simulink model "verify_Valve_Thermostatic_mdl"  (R2016b)
settings: Solver=ode45  StartTime=0.0  StopTime=100  MaxStep=1  RelTol=1e-3  EnableMultiTasking=on
libraries: carnot x2, simulink x1
settings Model: Creator=drhf  LastModifiedBy=drhf
settings DataIOCC: SaveFormat=Array  SignalLoggingSaveFormat=ModelDataLogs
settings OptimizationCC: ExpressionDepthLimit=2147483647  LifeSpan=inf
settings DebuggingCC: UnderspecifiedInitializationDetection=Classic  MergeDetectMultiDrivingBlocksExec=none  SolverPrmCheckMsg=warning  FcnCallInpInsideContextMsg=warning  StateNameClashWarn=warning  SFUnexpectedBacktrackingDiag=warning  SFNoUnconditionalDefaultTransitionDiag=warning  SFExecutionAtInitializationDiag=none
settings HardwareCC: ProdBitPerPointer=32  ProdBitPerSizeT=32  ProdBitPerPtrDiffT=32  ProdLargestAtomicFloat=None  ProdIntDivRoundTo=Undefined  ProdEndianess=Unspecified  ProdWordSize=32  ProdHWDeviceType=32-bit Generic
settings ModelReferenceCC: PropagateSignalLabelsOutOfModel=off
settings GRTTargetCC: TargetLangStandard=C89/C90 (ANSI)  GeneratePreprocessorConditionals=Disable all  CombineOutputUpdateFcns=off  GRTInterface=on
settings ConfigComp: CovMetricSettings=dw  CovHtmlReporting=on  CovSaveCumulativeToWorkspaceVar=on  CovSaveSingleToWorkspaceVar=on  CovExternalEMLEnable=off

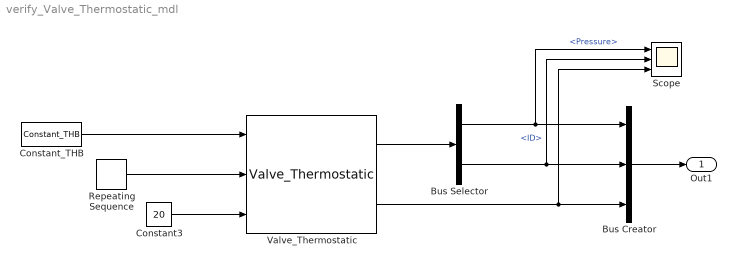
== system verify_Valve_Thermostatic_mdl ==
  Bus Creator : BusCreator  Inputs=3
  Bus Selector : BusSelector  OutputSignals=Pressure,ID
  Constant3 : Constant  Value=20
  Constant_THB : carnot/Source/Simple/Constant_THB  t=40  mdot=0.5  p=3e5  mID=Pressure Drop from Massflow  fluid=Water  mix=0  mix2=0  mix3=0  dia=0.02  hgt=0
  Repeating Sequence : simulink/Sources/Repeating Sequence  rep_seq_t=[0 50 100]  rep_seq_y=[15 25 15]
  Scope : Scope  NumInputPorts=3
  Valve_Thermostatic : carnot/Hydraulics/Valve_Thermostatic  p=4  op=0.5  bl=0.2  ts=1  dt_V=1  ART=linear  kvs=2  psi_0=0.04
  Out1 : Outport  SampleTime=5
  wires:
  Bus Creator/1 -> Out1/1
  Bus Selector/1 -> Bus Creator/1, Scope/1  "<Pressure>"
  Bus Selector/2 -> Bus Creator/2, Scope/2  "<ID>"
  Valve_Thermostatic/1 -> Bus Selector/1
  Repeating Sequence/1 -> Valve_Thermostatic/2
  Constant_THB/1 -> Valve_Thermostatic/1
  Constant3/1 -> Valve_Thermostatic/3
  Valve_Thermostatic/2 -> Bus Creator/3, Scope/3
